simulink model "heater"  (R2020b)
settings: Solver=VariableStepAuto  StartTime=0.0  StopTime=10.0  RelTol=1e-3
undefined symbols (not defined in the file): c, M, Mdot
settings Model: Creator=xinbo  LastModifiedBy=xinbo

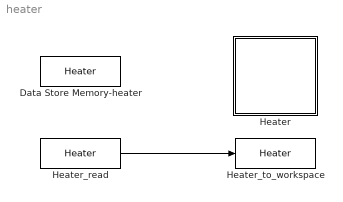
== system heater ==
  Data Store Memory-heater : DataStoreMemory  DataStoreName=Heater  ReadBeforeWriteMsg=warning  WriteAfterWriteMsg=warning  WriteAfterReadMsg=warning  ShowAdditionalParam=off
  Heater : Subsystem
      mask Display: image('$imagefile'); % Use "Edit Image" on toolstrip to change.
  Heater_read : DataStoreRead  DataStoreName=Heater
  Heater_to_workspace : ToWorkspace  VariableName=Heater  SampleTime=-1
      settings: Save2DSignal=2-D array (concatenate along first dimension)
  wires:
  Heater_read/1 -> Heater_to_workspace/1

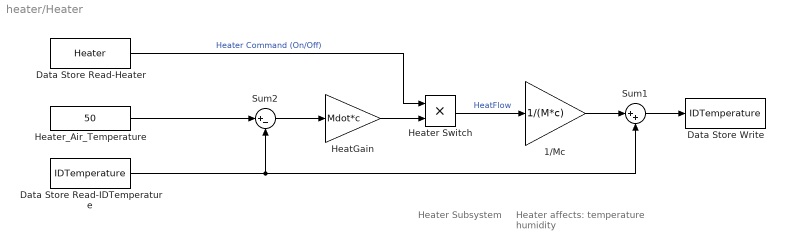
== system heater/Heater ==
  note: Heater affects:
      | temperature
      | humidity
  note: Heater Subsystem
  1/Mc : Gain  Gain=1/(M*c)  SaturateOnIntegerOverflow=on  OutDataTypeStr=Inherit: Same as input  ParamDataTypeStr=Inherit: Same as input
  Data Store Read-Heater : DataStoreRead  DataStoreName=Heater
  Data Store Read-IDTemperature : DataStoreRead  DataStoreName=IDTemperature
  Data Store Write : DataStoreWrite  DataStoreName=IDTemperature
  HeatGain : Gain  Gain=Mdot*c
  Heater Switch : Product  RndMeth=Zero
  Heater_Air_Temperature : Constant  Value=50
  Sum1 : Sum  Inputs=|++  InputSameDT=on  SaturateOnIntegerOverflow=on  OutDataTypeStr=Inherit: Same as first input
  Sum2 : Sum  Inputs=|+-
  wires:
  Data Store Read-Heater/1 -> Heater Switch/1  "Heater Command (On/Off)"
  Sum2/1 -> HeatGain/1
  Heater_Air_Temperature/1 -> Sum2/1
  HeatGain/1 -> Heater Switch/2
  Heater Switch/1 -> 1/Mc/1  "HeatFlow"
  1/Mc/1 -> Sum1/1
  Data Store Read-IDTemperature/1 -> Sum1/2, Sum2/2
  Sum1/1 -> Data Store Write/1
